simulink model "Controller"  (R2020a)
settings: Solver=VariableStepAuto  StartTime=0.0  StopTime=10  RelTol=1e-3
values from neighbouring files (symbols this model uses):
  Ki = 40    [MBD_W2_P3_Workspace.mat]
  Kp = 800    [MBD_W2_P3_Workspace.mat]
settings Model: DataDictionary=MBD_W2_P3_DataDictionary.sldd  Creator=Atri Mondal  LastModifiedBy=Atri Mondal
settings DataIOCC: SaveOutput=off  SaveTime=off

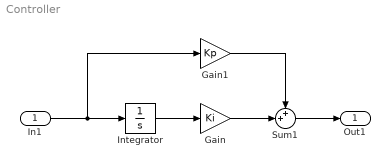
== system Controller ==
  In1 : Inport  OutDataTypeStr=double  PortDimensions=1  SampleTime=0
  Gain : Gain  Gain=Ki
  Gain1 : Gain  Gain=Kp
  Integrator : Integrator
  Sum1 : Sum  Inputs=++|
  Out1 : Outport  OutDataTypeStr=double  PortDimensions=1  SampleTime=0
  wires:
  Gain/1 -> Sum1/2
  Integrator/1 -> Gain/1
  In1/1 -> Integrator/1, Gain1/1
  Gain1/1 -> Sum1/1
  Sum1/1 -> Out1/1
